simulink model "semi_implicit_GSTA_const"  (R2018b)
settings: Solver=FixedStepAuto  StartTime=0.001  StopTime=7  FixedStep=0.001  MaxStep=0.1  RelTol=1e-3
InitFcn:
  | parameters_semi_gsta_const
model workspace: external: MAT-File (data not in the file)
values from neighbouring files (symbols this model uses):
  px = [1.5*sqrt(D)   2*1.1*D  1  1.5]    [parameters_semi_gsta_const.m]
  sample_plot = 0.01    [parameters_semi_gsta_const.m]
  sample_time = 0.05    [parameters_semi_gsta_const.m]
  v0 = -1    [parameters_semi_gsta_const.m]
  x0 = 1    [parameters_semi_gsta_const.m]
libraries: sdolib x1
settings Model: Creator=DING  LastModifiedBy=DNN
settings SolverCC: ZeroCrossAlgorithm=Adaptive
settings OptimizationCC: DefaultParameterBehavior=Inlined  EnhancedBackFolding=on  PassReuseOutputArgsAs=Individual arguments  MaxStackSize=64  OptimizeBlockOrder=speed  DifferentSizesBufferReuse=on
settings DebuggingCC: IgnoredZcDiagnostic=none  ParameterTunabilityLossMsg=error  UnderSpecifiedDimensionMsg=warning
settings HardwareCC: ProdBitPerPointer=32  ProdBitPerSizeT=32  ProdBitPerPtrDiffT=32  ProdLargestAtomicInteger=Long  ProdLargestAtomicFloat=Double  ProdWordSize=32  ProdHWDeviceType=ARM Compatible->ARM 11
settings SFSimCC: MATLABDynamicMemAlloc=off
settings RTWCC: SystemTargetFile=ert.tlc  TemplateMakefile=ert_default_tmf  GenerateReport=on  Toolchain=Catkin  IncludeHyperlinkInReport=on  LaunchReport=on  GenerateTraceInfo=on  GenerateTraceReport=on  GenerateTraceReportSl=on  GenerateTraceReportSf=on  GenerateTraceReportEml=on
settings CodeAppCC: ForceParamTrailComments=on  IgnoreCustomStorageClasses=off  OperatorAnnotations=on  SimulinkDataObjDesc=on  SFDataObjDesc=on  InsertBlockDesc=on
settings ERTTargetCC: ERTCustomFileTemplate=example_file_process.tlc

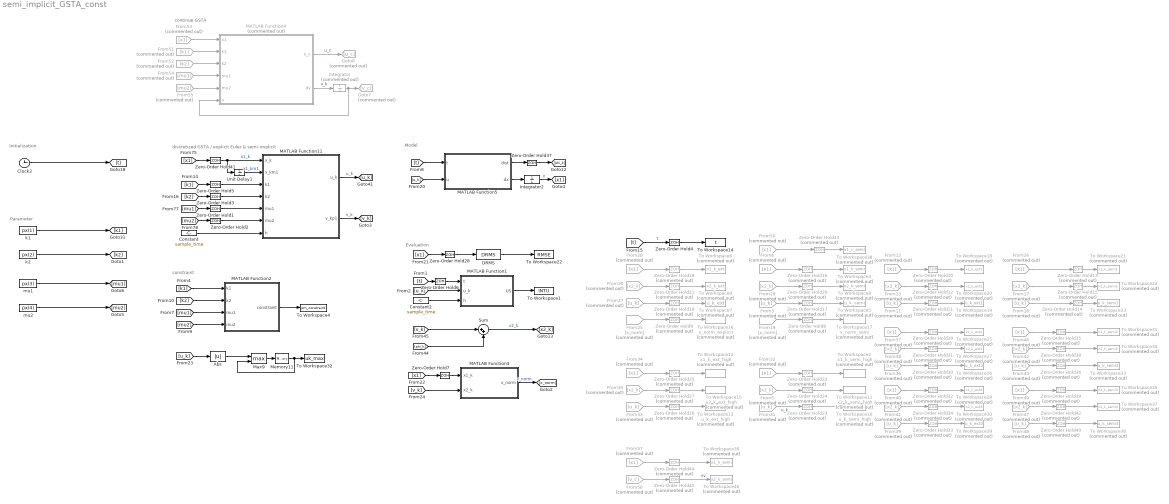
== system semi_implicit_GSTA_const ==
  note: discretized GSTA / explicit Euler & semi-implicit
  note: Initialization
  note: Evaluation
  note: Parameter
  note: Model
  note: constraint
  note: continue GSTA
  Abs : Abs
  Clock2 : Clock
  Constant : Constant  Value=sample_time  SampleTime=sample_time
  Constant2 : Constant  Value=sample_time  SampleTime=sample_time
  DRMS : sdolib/RMS Blocks/DRMS  Ts=sample_time
      settings: SourceProductBaseCode=SO
  From{3,11,18,27,31,33,36,39,43,48} (10 alike) : From  Commented=on  GotoTag=u_k
  From{6,12,26,28,32,34,37,40,46,49..50,53,57} (13 alike) : From  Commented=on  GotoTag=x1
  From{5,13,17,29..30,35,38,41..42,47} (10 alike) : From  Commented=on  GotoTag=x2_k
  From19 : From  Commented=on  GotoTag=x_norm
  From25 : From  Commented=on  GotoTag=x_norm
  From51 : From  Commented=on  GotoTag=k1
  From52 : From  Commented=on  GotoTag=k2
  From54 : From  Commented=on  GotoTag=mu1
  From55 : From  Commented=on  GotoTag=mu2
  From56 : From  Commented=on  GotoTag=v_c
  Goto7 : Goto  Commented=on  GotoTag=v_c
  Goto8 : Goto  Commented=on  GotoTag=u_c
  Integrator : Integrator  Commented=on  InitialCondition=v0
  Integrator2 : Integrator  InitialCondition=x0
  MATLAB Function1 : MATLAB Function  TreatAsAtomicUnit=on
  MATLAB Function11 : MATLAB Function  TreatAsAtomicUnit=on
  MATLAB Function2 : MATLAB Function  TreatAsAtomicUnit=on
  MATLAB Function3 : MATLAB Function  TreatAsAtomicUnit=on
  MATLAB Function4 : MATLAB Function  Commented=on  TreatAsAtomicUnit=on
  MATLAB Function5 : MATLAB Function  TreatAsAtomicUnit=on
  Max9 : MinMax  Function=max  Inputs=2
  Memory11 : Memory  InheritSampleTime=on
  Sum : Sum  Inputs=|++
  To Workspace1 : ToWorkspace  VariableName=INTU  SampleTime=-1
      settings: MaxDataPoints=1
  To Workspace10 : ToWorkspace  Commented=on  VariableName=u_k_semi_high  SampleTime=-1
  To Workspace11 : ToWorkspace  Commented=on  VariableName=x2_k_semi_high  SampleTime=-1
  To Workspace12 : ToWorkspace  Commented=on  VariableName=x1_k_ext_high  SampleTime=-1
  To Workspace13 : ToWorkspace  Commented=on  VariableName=u_k_ext_high  SampleTime=-1
  To Workspace14 : ToWorkspace  VariableName=t  SampleTime=-1
  To Workspace15 : ToWorkspace  Commented=on  VariableName=x2_k_ext_high  SampleTime=-1
  To Workspace16 : ToWorkspace  Commented=on  VariableName=x_norm_explicit  SampleTime=-1
  To Workspace17 : ToWorkspace  Commented=on  VariableName=x_norm_semi  SampleTime=-1
  To Workspace18 : ToWorkspace  Commented=on  VariableName=x1_k_ext1  SampleTime=-1
  To Workspace19 : ToWorkspace  Commented=on  VariableName=u_k_ext1  SampleTime=-1
  To Workspace2 : ToWorkspace  Commented=on  VariableName=x1_k_semi_high  SampleTime=-1
  To Workspace20 : ToWorkspace  Commented=on  VariableName=x2_k_ext1  SampleTime=-1
  To Workspace21 : ToWorkspace  Commented=on  VariableName=x1_k_semi1  SampleTime=-1
  To Workspace22 : ToWorkspace  VariableName=RMSE  SampleTime=-1
      settings: MaxDataPoints=1
  To Workspace23 : ToWorkspace  Commented=on  VariableName=u_k_semi1  SampleTime=-1
  To Workspace24 : ToWorkspace  Commented=on  VariableName=x2_k_semi1  SampleTime=-1
  To Workspace25 : ToWorkspace  Commented=on  VariableName=x1_k_ext2  SampleTime=-1
  To Workspace26 : ToWorkspace  Commented=on  VariableName=u_k_ext2  SampleTime=-1
  To Workspace27 : ToWorkspace  Commented=on  VariableName=x2_k_ext2  SampleTime=-1
  To Workspace28 : ToWorkspace  Commented=on  VariableName=x1_k_ext3  SampleTime=-1
  To Workspace29 : ToWorkspace  Commented=on  VariableName=u_k_ext3  SampleTime=-1
  To Workspace3 : ToWorkspace  Commented=on  VariableName=x1_k_semi  SampleTime=-1
  To Workspace30 : ToWorkspace  Commented=on  VariableName=x2_k_ext3  SampleTime=-1
  To Workspace31 : ToWorkspace  Commented=on  VariableName=x1_k_semi2  SampleTime=-1
  To Workspace32 : ToWorkspace  VariableName=uk_max  SampleTime=-1
      settings: MaxDataPoints=1
  To Workspace33 : ToWorkspace  Commented=on  VariableName=u_k_semi2  SampleTime=-1
  To Workspace34 : ToWorkspace  Commented=on  VariableName=x2_k_semi2  SampleTime=-1
  To Workspace35 : ToWorkspace  Commented=on  VariableName=x1_k_semi3  SampleTime=-1
  To Workspace36 : ToWorkspace  Commented=on  VariableName=u_k_semi3  SampleTime=-1
  To Workspace37 : ToWorkspace  Commented=on  VariableName=x2_k_semi3  SampleTime=-1
  To Workspace38 : ToWorkspace  Commented=on  VariableName=x1_c_semi  SampleTime=-1
  To Workspace39 : ToWorkspace  Commented=on  VariableName=x1_k_semi  SampleTime=-1
  To Workspace4 : ToWorkspace  VariableName=pm_constraint  SampleTime=-1
      settings: MaxDataPoints=1
  To Workspace40 : ToWorkspace  Commented=on  VariableName=x2_k_semi  SampleTime=-1
  To Workspace5 : ToWorkspace  Commented=on  VariableName=u_k_semi  SampleTime=-1
  To Workspace6 : ToWorkspace  Commented=on  VariableName=x1_k_ext  SampleTime=-1
  To Workspace7 : ToWorkspace  Commented=on  VariableName=u_k_ext  SampleTime=-1
  To Workspace8 : ToWorkspace  Commented=on  VariableName=x2_k_semi  SampleTime=-1
  To Workspace9 : ToWorkspace  Commented=on  VariableName=x2_k_ext  SampleTime=-1
  Unit Delay1 : UnitDelay  InitialCondition=1  SampleTime=-1
  Zero-Order Hold{1..3,5..7,28,37,41} (9 alike) : ZeroOrderHold  SampleTime=sample_time
  Zero-Order Hold{8..27,29..36,38..40,42..45} (35 alike) : ZeroOrderHold  Commented=on  SampleTime=sample_plot
  Zero-Order Hold4 : ZeroOrderHold  SampleTime=sample_plot
  k1 : Constant  Value=px(1)
  k2 : Constant  Value=px(2)
  mu1 : Constant  Value=px(3)
  mu2 : Constant  Value=px(4)
  wires:
  [mu1] -> Zero-Order Hold1/1
  [mu2] -> Zero-Order Hold2/1
  MATLAB Function11/2(v_kp1) -> [v_k]  "v_k"
  Constant/1 -> MATLAB Function11/7(h)
  Zero-Order Hold1/1 -> MATLAB Function11/5(mu1)
  Zero-Order Hold2/1 -> MATLAB Function11/6(mu2)
  MATLAB Function11/1(u_k) -> [u_k]  "u_k"
  [t] -> Zero-Order Hold4/1  "t"
  From3/1 -> Zero-Order Hold17/1
  [t] -> MATLAB Function5/1(t)
  Integrator2/1 -> [x1]  "x"
  MATLAB Function5/2(dx) -> Integrator2/1
  MATLAB Function5/1(dist) -> Zero-Order Hold37/1
  Zero-Order Hold3/1 -> MATLAB Function11/4(k2)
  Zero-Order Hold5/1 -> MATLAB Function11/3(k1)
  [k1] -> Zero-Order Hold5/1
  [k2] -> Zero-Order Hold3/1
  k1/1 -> [k1]
  k2/1 -> [k2]
  mu2/1 -> [mu2]
  mu1/1 -> [mu1]
  [x1] -> Zero-Order Hold28/1
  DRMS/1 -> To Workspace22/1
  Zero-Order Hold41/1 -> MATLAB Function11/1(x_k), Unit Delay1/1  "x1_k"
  [x1] -> Zero-Order Hold41/1
  [u_k] -> MATLAB Function1/2(u_k)
  MATLAB Function1/1(US) -> To Workspace1/1
  Constant2/1 -> MATLAB Function1/3(h)
  Clock2/1 -> [t]
  Zero-Order Hold4/1 -> To Workspace14/1
  Zero-Order Hold16/1 -> To Workspace3/1
  Zero-Order Hold17/1 -> To Workspace5/1
  Zero-Order Hold19/1 -> To Workspace7/1
  From28/1 -> Zero-Order Hold18/1
  Zero-Order Hold18/1 -> To Workspace6/1
  From27/1 -> Zero-Order Hold19/1
  Zero-Order Hold20/1 -> To Workspace8/1
  From29/1 -> Zero-Order Hold20/1
  Zero-Order Hold21/1 -> To Workspace9/1
  From30/1 -> Zero-Order Hold21/1
  From32/1 -> Zero-Order Hold22/1
  Zero-Order Hold23/1 -> To Workspace10/1
  From5/1 -> Zero-Order Hold24/1
  From31/1 -> Zero-Order Hold23/1  "u_k"
  Zero-Order Hold24/1 -> To Workspace11/1
  Zero-Order Hold22/1 -> To Workspace2/1
  From35/1 -> Zero-Order Hold27/1
  Zero-Order Hold25/1 -> To Workspace12/1
  Zero-Order Hold26/1 -> To Workspace13/1
  From34/1 -> Zero-Order Hold25/1
  Zero-Order Hold27/1 -> To Workspace15/1
  From33/1 -> Zero-Order Hold26/1
  Zero-Order Hold28/1 -> DRMS/1
  Unit Delay1/1 -> MATLAB Function11/2(x_km1)  "x1_km1"
  Zero-Order Hold37/1 -> [phi_k]
  Sum/1 -> [x2_k]  "x2_k"
  [v_k] -> Sum/1
  [phi_k] -> Sum/2
  [t] -> Zero-Order Hold6/1
  Zero-Order Hold6/1 -> MATLAB Function1/1(t)
  [k1] -> MATLAB Function2/1(k1)
  MATLAB Function2/1(constraint) -> To Workspace4/1
  [mu2] -> MATLAB Function2/4(mu2)
  [mu1] -> MATLAB Function2/3(mu1)
  [k2] -> MATLAB Function2/2(k2)
  Max9/1 -> Memory11/1
  [u_k] -> Abs/1
  Abs/1 -> Max9/1
  Memory11/1 -> To Workspace32/1, Max9/2
  [u_k] -> MATLAB Function5/2(u)
  [v_k] -> MATLAB Function3/2(x2_k)
  [x1] -> Zero-Order Hold7/1
  Zero-Order Hold7/1 -> MATLAB Function3/1(x1_k)
  MATLAB Function3/1(x_norm) -> [x_norm]  "x_norm"
  From19/1 -> Zero-Order Hold8/1
  Zero-Order Hold8/1 -> To Workspace17/1
  Zero-Order Hold9/1 -> To Workspace16/1
  From25/1 -> Zero-Order Hold9/1
  From12/1 -> Zero-Order Hold10/1
  Zero-Order Hold12/1 -> To Workspace20/1
  From13/1 -> Zero-Order Hold12/1
  From11/1 -> Zero-Order Hold11/1
  Zero-Order Hold11/1 -> To Workspace19/1
  Zero-Order Hold10/1 -> To Workspace18/1
  Zero-Order Hold13/1 -> To Workspace21/1
  From26/1 -> Zero-Order Hold13/1
  Zero-Order Hold15/1 -> To Workspace24/1
  Zero-Order Hold14/1 -> To Workspace23/1
  From17/1 -> Zero-Order Hold15/1
  From18/1 -> Zero-Order Hold14/1
  Zero-Order Hold29/1 -> To Workspace25/1
  From38/1 -> Zero-Order Hold31/1
  Zero-Order Hold30/1 -> To Workspace26/1
  Zero-Order Hold31/1 -> To Workspace27/1
  From36/1 -> Zero-Order Hold30/1
  From37/1 -> Zero-Order Hold29/1
  From39/1 -> Zero-Order Hold33/1
  Zero-Order Hold34/1 -> To Workspace30/1
  From40/1 -> Zero-Order Hold32/1
  From41/1 -> Zero-Order Hold34/1
  Zero-Order Hold33/1 -> To Workspace29/1
  Zero-Order Hold32/1 -> To Workspace28/1
  Zero-Order Hold38/1 -> To Workspace34/1
  From43/1 -> Zero-Order Hold36/1
  From46/1 -> Zero-Order Hold35/1
  Zero-Order Hold35/1 -> To Workspace31/1
  Zero-Order Hold36/1 -> To Workspace33/1
  From42/1 -> Zero-Order Hold38/1
  From47/1 -> Zero-Order Hold42/1
  Zero-Order Hold40/1 -> To Workspace36/1
  From49/1 -> Zero-Order Hold39/1
  Zero-Order Hold39/1 -> To Workspace35/1
  From48/1 -> Zero-Order Hold40/1
  Zero-Order Hold42/1 -> To Workspace37/1
  From6/1 -> Zero-Order Hold16/1
  From50/1 -> Zero-Order Hold43/1
  Zero-Order Hold43/1 -> To Workspace38/1
  From53/1 -> MATLAB Function4/1(x1)
  From51/1 -> MATLAB Function4/2(k1)
  From52/1 -> MATLAB Function4/3(k2)
  MATLAB Function4/1(u_c) -> Goto8/1  "u_c"
  From55/1 -> MATLAB Function4/5(mu2)
  From54/1 -> MATLAB Function4/4(mu1)
  MATLAB Function4/2(dv) -> Integrator/1  "v_k"
  From57/1 -> Zero-Order Hold44/1
  From56/1 -> Zero-Order Hold45/1
  Zero-Order Hold45/1 -> To Workspace40/1  "vv"
  Zero-Order Hold44/1 -> To Workspace39/1
  Integrator/1 -> MATLAB Function4/6(v), Goto7/1

== matlab function semi_implicit_GSTA_const/MATLAB Function2 ==
  data: k1 input; k2 input; mu1 input; mu2 input; constraint output
function constraint = pm_constraint(k1, k2, mu1, mu2)

h=0.05;
if k1>(2-4*h^2*k2*mu2^2)/(h*mu2)
    constraint=1;
else    
    constraint=0;
end

end

== matlab function semi_implicit_GSTA_const/MATLAB Function1 ==
  data: t input; US output; u_k input; h input
function US = EVAU(t, u_k, h)
persistent sum_uk_initial

if isempty(sum_uk_initial)
    sum_uk_initial=0;
    sum_uk=sum_uk_initial;
else
    if t<=0.5
        sum_uk=sum_uk_initial+1*abs(u_k);
    else
        sum_uk=sum_uk_initial+abs(u_k);
    end
    sum_uk_initial=sum_uk;
end

US=sum_uk/(10/h);

end

== matlab function semi_implicit_GSTA_const/MATLAB Function3 ==
  data: x1_k input; x2_k input; x_norm output
function x_norm = calcu_xnorm(x1_k, x2_k)

x_norm=sqrt(x1_k^2+x2_k^2);

end

== matlab function semi_implicit_GSTA_const/MATLAB Function4 ==
  data: x1 input; k1 input; k2 input; mu1 input; mu2 input; v input; u_c output; dv output
function [u_c, dv] = GSTA(x1, k1, k2, mu1, mu2, v)

phi1 = mu1*abs(x1)^0.5*sign(x1)+mu2*x1;

phi2 = 0.5*mu1^2*sign(x1)+1.5*mu1*mu2*abs(x1)^0.5*sign(x1)+mu2^2*x1;

dv = -k2*phi2;

u_c = -k1*phi1 + k2*v;

end

== matlab function semi_implicit_GSTA_const/MATLAB Function5 ==
  data: dist output; dx output; t input; u input
function [dist,dx]= Dynamic_Model(t,u)

% fx=0.6*sin(x)+0.7*x^2-1.5*x;
% dxt=0.8*cos(x)*x+0.05*cos(3*t)+0.08*sin(t);
% dx=fx+dxt+u;

dist=0;
% dist=5*cos(t);
% dist=1.2*cos(2*t)+0.4*sqrt(10)*cos(sqrt(10)*t);

dx=u+dist;

end

== matlab function semi_implicit_GSTA_const/MATLAB Function11 ==
  data: x_k input; x_km1 input; k1 input; k2 input; mu1 input; mu2 input; h input; u_k output; v_kp1 output
function [u_k, v_kp1] = GSTA(x_k, x_km1, k1, k2, mu1, mu2, h)

persistent v_k

lam_sum = -k1 * (mu1*abs(x_k)^-0.5 + mu2);
lam_multi = k2 * (0.5*mu1^2 * abs(x_k)^-1 + 1.5*mu1*mu2*abs(x_k)^-0.5 + mu2^2);
lam_sum_m1 = -k1 * (mu1*abs(x_km1)^-0.5 + mu2);
lam_multi_m1 = k2 * (0.5*mu1^2 * abs(x_km1)^-1 + 1.5*mu1*mu2*abs(x_km1)^-0.5 + mu2^2);

% abs(x_k) <=1e-6 x_k==0
if x_k==0
    q_sum = 0;
    q_sum_m1 = 0;
    q_multi_m1 = 0;
else
    % explicit Euler
%     q_sum = 2 + h*lam_sum; 
%     q_sum_m1 = 2 + h*lam_sum_m1; 
%     q_multi_m1 = 1 + h*lam_sum_m1 + h^2*lam_multi_m1;

    % semi-impliict
    q_sum = (2 - h * lam_sum ) / (1 - h * lam_sum + h^2 * lam_multi ); 
    q_sum_m1 = (2 - h * lam_sum_m1 ) / (1 - h * lam_sum_m1 + h^2 * lam_multi_m1 ); 
    q_multi_m1 = 1 / (1 - h * lam_sum_m1 + h^2 * lam_multi_m1 );
end

u1_k = q_sum - 1;    % u1_k=q1+q2-1;
u1_k_m1 = q_sum_m1 - 1;    % u1_k=q1+q2-1;
u2_k_m1 = 1/h * (u1_k_m1 - q_multi_m1);   % u2_k=1/h*(u1_k-q1*q2);

if isempty(v_k)
    v_k=-1;
    v_kp1=v_k;
else
    v_kp1 = v_k + u2_k_m1 * x_km1;
    v_k=v_kp1;
end

u_k = 1/h * ( - x_k + u1_k * x_k ) + v_kp1;

end
